simulink model "lab4_S6_7_8_estimation_control_yaw"  (R2024b)
settings: Solver=ode23  StartTime=0.0  StopTime=sIn.simulation_time  RelTol=1e-3
undefined symbols (not defined in the file): chassis, DiscIntNeverNeededParam, drv, feedback, filter, gbox, sens, sIn, wheel
settings Model: Creator=Nihal  LastModifiedBy=pries

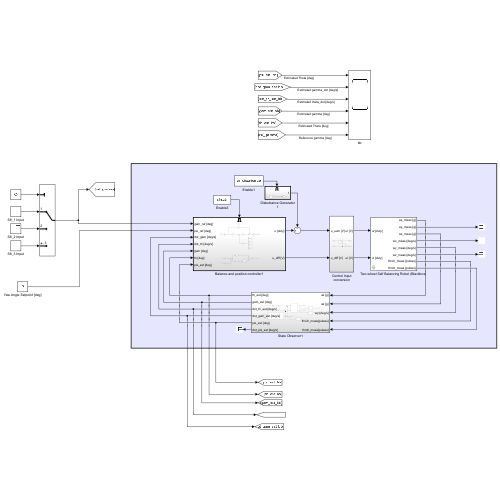
[thumbnail: Simulink's stored preview of the top-level diagram]
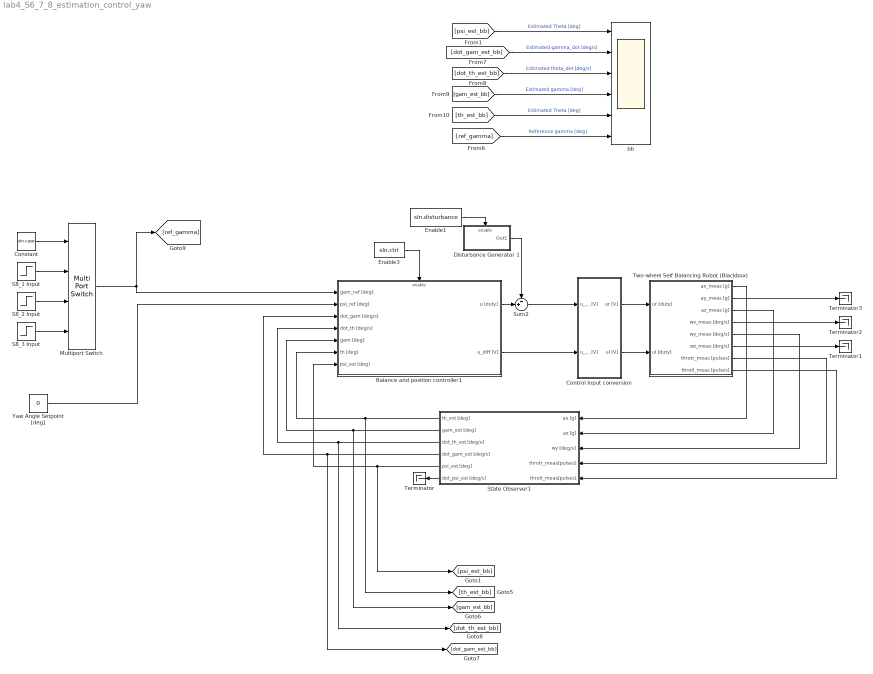
== system lab4_S6_7_8_estimation_control_yaw ==
  Balance and position controller1 : Subsystem
  Constant : Constant  Value=sIn.case
  Control Input conversion : Subsystem
  Disturbance Generator 1 : Subsystem  TreatAsAtomicUnit=on
  Enable1 : Constant  Value=sIn.disturbance
  Enable3 : Constant  Value=sIn.ctrl
  Multiport Switch : MultiPortSwitch  SaturateOnIntegerOverflow=off  InputSameDT=off
  S8_1 Input : Step  Time=0  After=0  SampleTime=0
  S8_2 Input : Step  Time=0  After=(0.1/wheel.r) *rad2deg  SampleTime=0
  S8_3 Input : Step  Time=0  After=(0.1/wheel.r) *rad2deg  SampleTime=0
  State Observer1 : Subsystem
  Sum2 : Sum  Inputs=-+|
  Terminator{,1..3} (4 alike) : Terminator
  "Two-wheel Self Balancing Robot (Blackbox) " : Subsystem  mask(Balancing robot (longitudinal + lateral dynamics)){initState=sIn.bb_ic, Ts=0.01}
      mask prompts: initState "Initial state [gam(0), psi(0), th(0), dot_gam(0), dot_psi(0), dot_th(0)]'"; Ts "Sample time:"
      mask help:
      | Balancing robot dynamic model.
      | Includes both the longitudinal and lateral (yaw) dynamics.
      mask init:
      | %% General parameters and conversion gains
      | 
      | %   gravity acc [m/s^2]
      | g = 9.81;
      | 
      | %   conversion gains
      | rpm2rads = 2*pi/60;         %   [rpm]   -> [rad/s]
      | rads2rpm = 60/2/pi;         %   [rad/s] -> [rpm]
      | rpm2degs = 360/60;          %   [rpm]   -> [deg/s]
      | degs2rpm = 60/360;          %   [deg/s] -> [rpm]
      | deg2rad = pi/180;           %   [deg]   -> [rad]
      | rad2deg = 180/pi;           %   [rad]   -> [deg]
      | g2ms2 = g;                  %   [acc_g] -> [m/s^2]
      | ms22g = 1/g;                %   [m/s^2] -> [acc_g]
      | ozin2Nm = 0.706e-2;         %   [oz*inch] -> [N*m]
      | 
      | 
      | %%  Battery data
      | 
      | %   electrical data
      | batt.UN = 11.1;     %   nominal voltage
      | 
      | 
      | %%  H-bridge PWM voltage driver
      | 
      | drv.Vbus = batt.UN;                     %   H-bridge DC bus voltage  
      | drv.pwm.bits = 8;                       %   PWM resolution [bits]
      | drv.pwm.levels = 2^drv.pwm.bits;        %   PWM levels
      | drv.pwm.Fs = 490;                       %   PWM frequency
      | drv.dutymax = drv.pwm.levels-1;         %   max duty cycle code
      | drv.duty2V = drv.Vbus/drv.dutymax;      %   duty cycle code (0-255) to voltage
      | drv.V2duty = drv.dutymax/drv.Vbus;      %   voltage to duty cycle code (0-255)
      | 
      | 
      | %%  Gearbox data 
      | 
      | gbox.N = 30;            %   reduction ratio
      | 
      | 
      | %%  Sensors data - Hall-effect encoder
      | 
      | %   Hall-effect encoder
      | sens.enc.ppr = 16*4;    %   pulses per rotation at motor side (w/ quadrature decoding)
      | sens.enc.pulse2deg = 360/sens.enc.ppr;
      | sens.enc.pulse2rad = 2*pi/sens.enc.ppr;
      | sens.enc.deg2pulse = sens.enc.ppr/360;
      | sens.enc.rad2pulse = sens.enc.ppr/2/pi;
      | 
      | 
      | %%  Sensors data - MPU6050 (accelerometer + gyro)
      | 
      | %   center of mass (CoM) position
      | sens.mpu.xb = 0;
      | sens.mpu.yb = 0;
      | sens.mpu.zb = 13.5e-3;
      | 
      | %       MPU6050 embedded accelerometer specs
      | sens.mpu.acc.bits = 16;
      | sens.mpu.acc.fs_g = 16;                                                         %   full-scale in "g" units
      | sens.mpu.acc.fs = sens.mpu.acc.fs_g * g2ms2;                                    %   full-scale in [m/s^2] 
      | sens.mpu.acc.g2LSB = floor(2^(sens.mpu.acc.bits-1)/sens.mpu.acc.fs_g);          %   sensitivity [LSB/g]
      | sens.mpu.acc.ms22LSB = sens.mpu.acc.g2LSB * ms22g;                              %   sensitvity [LSB/(m/s^2)]
      | sens.mpu.acc.LSB2g = sens.mpu.acc.fs_g/2^(sens.mpu.acc.bits-1);                 %   output quantization step [g/LSB]
      | sens.mpu.acc.LSB2ms2 = sens.mpu.acc.LSB2g * g2ms2;                              %   output quantization step [ms2/LSB]
      | sens.mpu.acc.bw = 94;                                                           %   output low-pass filter bandwidth
      | sens.mpu.acc.noisestd = 400e-6*sqrt(100);                                       %   output noise std [g-rms]
      | sens.mpu.acc.noisevar = sens.mpu.acc.noisestd^2;                                %   output noise var [g^2]
      | 
      | %       MPU6050 embdedded gyroscope specs
      | sens.mpu.gyro.bits = 16;
      | sens.mpu.gyro.fs_degs = 250;                                                    %   full scale in [deg/s (dps)]
      | sens.mpu.gyro.fs = sens.mpu.gyro.fs_degs * deg2rad;                             %   full scale in [rad/s]
      | sens.mpu.gyro.degs2LSB = floor(2^(sens.mpu.gyro.bits-1)/sens.mpu.gyro.fs_degs);	%   sensitivity [LSB/degs]
      | sens.mpu.gyro.rads2LSB = sens.mpu.gyro.degs2LSB * rad2deg;                      %   sensitivity [LSB/rads] 
      | sens.mpu.gyro.LSB2degs = sens.mpu.gyro.fs_degs/2^(sens.mpu.gyro.bits-1);        %   output quantization step [degs/LSB]
      | sens.mpu.gyro.LSB2rads = sens.mpu.gyro.LSB2degs * deg2rad;                      %   output quantization step [rads/LSB]
      | sens.mpu.gyro.bw = 98;                                                          %   output low-pass filter bandwidth
      | sens.mpu.gyro.noisestd = 5e-3*sqrt(100);                                        %   output noise std [degs-rms]
      | sens.mpu.gyro.noisevar = sens.mpu.acc.noisestd ^2;                              %   output noise var [degs^2]
      mask Help:
      | Riccardo Antonello (antonello@dei.unipd.it)
      | 
      | May 19, 2020
      | 
      | Dept. of Information Engineering, University of Padova
  Yaw Angle Setpoint [deg] : Constant  Value=0
  bb : Scope  NumInputPorts=6
  wires:
  Multiport Switch/1 -> [ref_gamma], Balance and position controller1/1(gam_ref [deg])
  "Two-wheel Self Balancing Robot (Blackbox) "/1(ax_meas [g]) -> State Observer1/1(ax [g])
  "Two-wheel Self Balancing Robot (Blackbox) "/3(az_meas [g]) -> State Observer1/2(az [g])
  "Two-wheel Self Balancing Robot (Blackbox) "/5(wy_meas [deg/s]) -> State Observer1/3(wy [deg/s])
  State Observer1/4(dot_gam_est [deg/s]) -> [dot_gam_est_bb], Balance and position controller1/3(dot_gam [deg/s])
  State Observer1/2(gam_est [deg]) -> [gam_est_bb], Balance and position controller1/5(gam [deg])
  State Observer1/1(th_est [deg]) -> [th_est_bb], Balance and position controller1/6(th [deg])
  State Observer1/3(dot_th_est [deg/s]) -> [dot_th_est_bb], Balance and position controller1/4(dot_th [deg/s])
  [dot_th_est_bb] -> bb/3  "Estimated theta_dot [deg/s]"
  [gam_est_bb] -> bb/4  "Estimated gamma [deg]"
  [ref_gamma] -> bb/6  "Reference gamma [deg]"
  [th_est_bb] -> bb/5  "Estimated Theta [deg]"
  [dot_gam_est_bb] -> bb/2  "Estimated gamma_dot [deg/s]"
  S8_1 Input/1 -> Multiport Switch/2
  S8_2 Input/1 -> Multiport Switch/3
  Constant/1 -> Multiport Switch/1
  S8_3 Input/1 -> Multiport Switch/4
  Enable1/1 -> Disturbance Generator 1/Enable
  Balance and position controller1/1(u [duty]) -> Sum2/2
  Sum2/1 -> Control Input conversion/1(u_sum [V])
  Disturbance Generator 1/1(Out1) -> Sum2/1
  Enable3/1 -> Balance and position controller1/Enable
  State Observer1/5(psi_est [deg]) -> Balance and position controller1/7(psi_est [deg]), [psi_est_bb]
  State Observer1/6(dot_psi_est [deg/s]) -> Terminator/1
  Yaw Angle Setpoint [deg]/1 -> Balance and position controller1/2(psi_ref [deg])
  Control Input conversion/2(ul [V]) -> "Two-wheel Self Balancing Robot (Blackbox) "/2(ul [duty])
  Control Input conversion/1(ur [V]) -> "Two-wheel Self Balancing Robot (Blackbox) "/1(ur [duty])
  Balance and position controller1/2(u_diff [V]) -> Control Input conversion/2(u_diff [V])
  "Two-wheel Self Balancing Robot (Blackbox) "/8(throtl_meas [pulses]) -> State Observer1/5(throtl_meas[pulses])
  "Two-wheel Self Balancing Robot (Blackbox) "/7(throtr_meas [pulses]) -> State Observer1/4(throtr_meas[pulses])
  "Two-wheel Self Balancing Robot (Blackbox) "/6(wz_meas [deg/s]) -> Terminator1/1
  "Two-wheel Self Balancing Robot (Blackbox) "/4(wx_meas [deg/s]) -> Terminator2/1
  "Two-wheel Self Balancing Robot (Blackbox) "/2(ay_meas [g]) -> Terminator3/1
  [psi_est_bb] -> bb/1  "Estimated Theta [deg]"

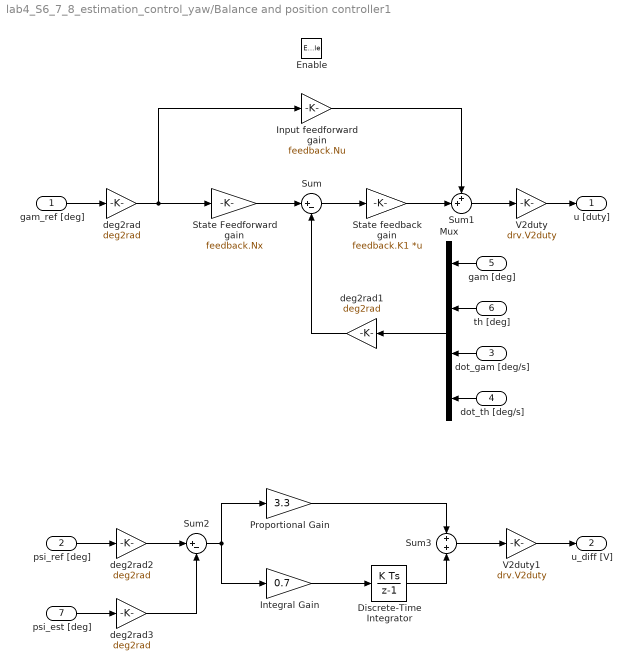
== system lab4_S6_7_8_estimation_control_yaw/Balance and position controller1 ==
  gam_ref [deg] : Inport
  psi_ref [deg] : Inport  Port=2
  dot_gam [deg/s] : Inport  Port=3
  dot_th [deg/s] : Inport  Port=4
  gam [deg] : Inport  Port=5
  th [deg] : Inport  Port=6
  psi_est [deg] : Inport  Port=7
  Enable : EnablePort
  Discrete-Time Integrator : DiscreteIntegrator  SampleTime=-1  ICPrevOutput=DiscIntNeverNeededParam  ICPrevScaledInput=DiscIntNeverNeededParam
  Input feedforward gain : Gain  Gain=feedback.Nu
  Integral Gain : Gain  Gain=0.7
  Mux : Mux
  Proportional Gain : Gain  Gain=3.3
  State Feedforward gain : Gain  Gain=feedback.Nx
  State feedback gain : Gain  Gain=feedback.K1  Multiplication=Matrix(K*u)
  Sum : Sum  Inputs=|+-
  Sum1 : Sum  Inputs=++|
  Sum2 : Sum  Inputs=|+-
  Sum3 : Sum  Inputs=+|+
  V2duty : Gain  Gain=drv.V2duty
  V2duty1 : Gain  Gain=drv.V2duty
  deg2rad{,1..3} (4 alike) : Gain  Gain=deg2rad
  u [duty] : Outport  OutputWhenDisabled=reset  InitialOutput=0
  u_diff [V] : Outport  Port=2  OutputWhenDisabled=reset  InitialOutput=0
  wires:
  gam_ref [deg]/1 -> deg2rad/1
  deg2rad/1 -> Input feedforward gain/1, State Feedforward gain/1
  State Feedforward gain/1 -> Sum/1
  deg2rad1/1 -> Sum/2
  Mux/1 -> deg2rad1/1
  gam [deg]/1 -> Mux/1
  dot_th [deg/s]/1 -> Mux/4
  dot_gam [deg/s]/1 -> Mux/3
  th [deg]/1 -> Mux/2
  Sum/1 -> State feedback gain/1
  State feedback gain/1 -> Sum1/2
  Input feedforward gain/1 -> Sum1/1
  Sum1/1 -> V2duty/1
  V2duty/1 -> u [duty]/1
  psi_ref [deg]/1 -> deg2rad2/1
  psi_est [deg]/1 -> deg2rad3/1
  deg2rad2/1 -> Sum2/1
  deg2rad3/1 -> Sum2/2
  Integral Gain/1 -> Discrete-Time Integrator/1
  Sum2/1 -> Integral Gain/1, Proportional Gain/1
  Proportional Gain/1 -> Sum3/1
  Discrete-Time Integrator/1 -> Sum3/2
  Sum3/1 -> V2duty1/1
  V2duty1/1 -> u_diff [V]/1

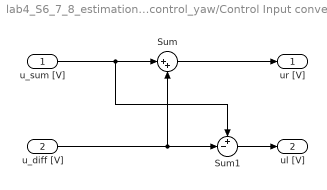
== system lab4_S6_7_8_estimation_control_yaw/Control Input conversion ==
  u_sum [V] : Inport
  u_diff [V] : Inport  Port=2
  Sum : Sum  Inputs=|++
  Sum1 : Sum  Inputs=+-|
  ur [V] : Outport
  ul [V] : Outport  Port=2
  wires:
  u_sum [V]/1 -> Sum/1, Sum1/1
  Sum/1 -> ur [V]/1
  u_diff [V]/1 -> Sum/2, Sum1/2
  Sum1/1 -> ul [V]/1

== system lab4_S6_7_8_estimation_control_yaw/Disturbance Generator 1 ==
  Enable : EnablePort
  Step : Step  Time=10  After=5/drv.duty2V  SampleTime=0
  Out1 : Outport  OutputWhenDisabled=reset  InitialOutput=0
  wires:
  Step/1 -> Out1/1

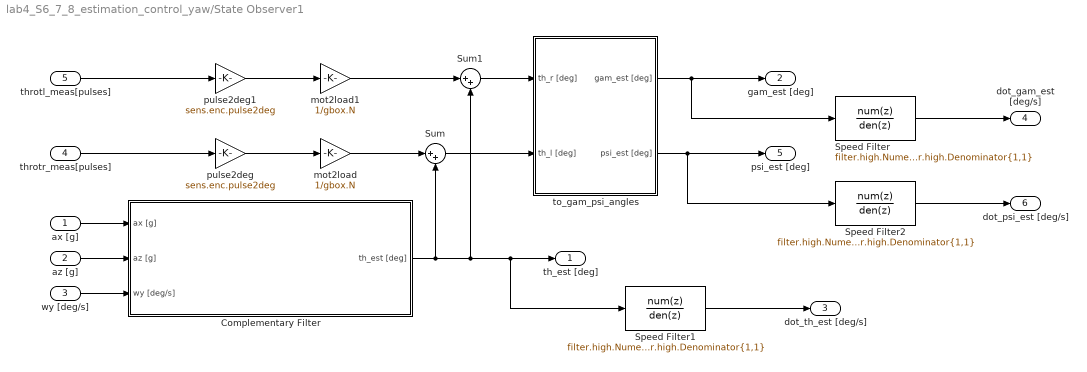
== system lab4_S6_7_8_estimation_control_yaw/State Observer1 ==
  ax [g] : Inport
  az [g] : Inport  Port=2
  wy [deg/s] : Inport  Port=3
  throtr_meas[pulses] : Inport  Port=4
  throtl_meas[pulses] : Inport  Port=5
  Complementary Filter : Subsystem
  Speed Filter : DiscreteFilter  Numerator=filter.high.Numerator{1,1}  Denominator=filter.high.Denominator{1,1}
  Speed Filter1 : DiscreteFilter  Numerator=filter.high.Numerator{1,1}  Denominator=filter.high.Denominator{1,1}
  Speed Filter2 : DiscreteFilter  Numerator=filter.high.Numerator{1,1}  Denominator=filter.high.Denominator{1,1}
  Sum : Sum  Inputs=|++
  Sum1 : Sum  Inputs=|++
  mot2load : Gain  Gain=1/gbox.N
  mot2load1 : Gain  Gain=1/gbox.N
  pulse2deg : Gain  Gain=sens.enc.pulse2deg
  pulse2deg1 : Gain  Gain=sens.enc.pulse2deg
  to_gam_psi_angles : Subsystem
  th_est [deg] : Outport
  gam_est [deg] : Outport  Port=2
  dot_th_est [deg/s] : Outport  Port=3
  dot_gam_est [deg/s] : Outport  Port=4
  psi_est [deg] : Outport  Port=5
  dot_psi_est [deg/s] : Outport  Port=6
  wires:
  wy [deg/s]/1 -> Complementary Filter/3(wy [deg/s])
  az [g]/1 -> Complementary Filter/2(az [g])
  ax [g]/1 -> Complementary Filter/1(ax [g])
  Complementary Filter/1(th_est [deg]) -> Sum/2, Sum1/2, Speed Filter1/1, th_est [deg]/1
  throtr_meas[pulses]/1 -> pulse2deg/1
  pulse2deg/1 -> mot2load/1
  mot2load/1 -> Sum/1
  Speed Filter1/1 -> dot_th_est [deg/s]/1
  Speed Filter/1 -> dot_gam_est [deg/s]/1
  mot2load1/1 -> Sum1/1
  pulse2deg1/1 -> mot2load1/1
  throtl_meas[pulses]/1 -> pulse2deg1/1
  Sum/1 -> to_gam_psi_angles/2(th_l [deg])
  Sum1/1 -> to_gam_psi_angles/1(th_r [deg])
  to_gam_psi_angles/1(gam_est [deg]) -> Speed Filter/1, gam_est [deg]/1
  to_gam_psi_angles/2(psi_est [deg]) -> Speed Filter2/1, psi_est [deg]/1
  Speed Filter2/1 -> dot_psi_est [deg/s]/1

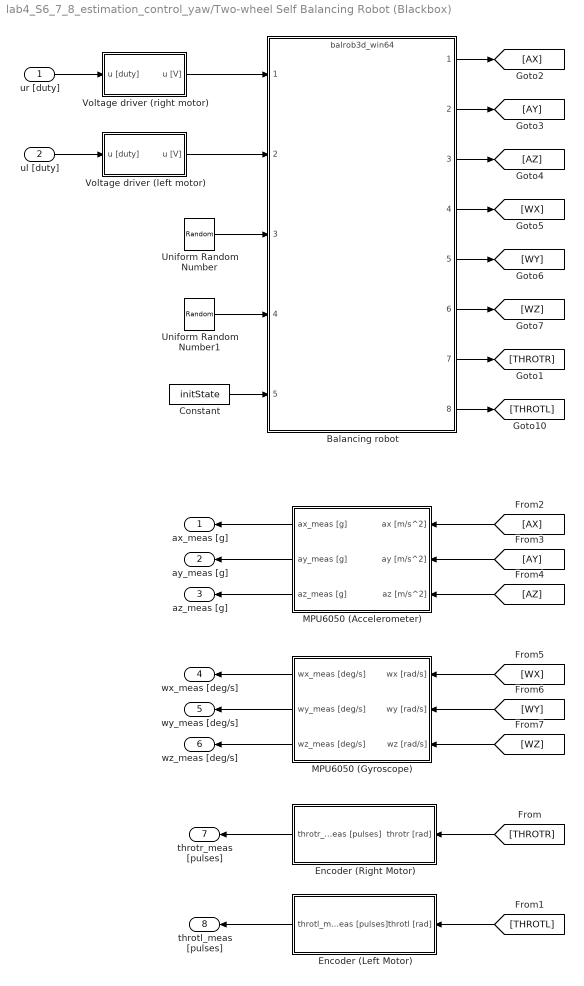
== system lab4_S6_7_8_estimation_control_yaw/Two-wheel Self Balancing Robot (Blackbox)  ==
  ur [duty] : Inport
  ul [duty] : Inport  Port=2
  Balancing robot : ModelReference  ModelNameDialog=balrob3d_win64.slxp  ModelReferenceVersion=1.741  CopyOfModelProtected=on
  Constant : Constant  Value=initState
  Encoder (Left Motor) : Subsystem
  Encoder (Right Motor) : Subsystem
  MPU6050 (Accelerometer) : Subsystem
  MPU6050 (Gyroscope) : Subsystem
  Uniform Random Number : UniformRandomNumber  Minimum=0.7  Maximum=1.3  SampleTime=1
  Uniform Random Number1 : UniformRandomNumber  Minimum=0.7  Maximum=1.3  Seed=10  SampleTime=1
  Voltage driver (left motor) : Subsystem
  Voltage driver (right motor) : Subsystem
  ax_meas [g] : Outport
  ay_meas [g] : Outport  Port=2
  az_meas [g] : Outport  Port=3
  wx_meas [deg/s] : Outport  Port=4
  wy_meas [deg/s] : Outport  Port=5
  wz_meas [deg/s] : Outport  Port=6
  throtr_meas [pulses] : Outport  Port=7
  throtl_meas [pulses] : Outport  Port=8
  wires:
  ur [duty]/1 -> Voltage driver (right motor)/1(u [duty])
  [WX] -> MPU6050 (Gyroscope)/1(wx [rad/s])
  Balancing robot/2 -> [AY]
  Balancing robot/4 -> [WX]
  Balancing robot/8 -> [THROTL]
  Balancing robot/1 -> [AX]
  [THROTL] -> Encoder (Left Motor)/1(throtl [rad])
  Balancing robot/6 -> [WZ]
  Balancing robot/7 -> [THROTR]
  Balancing robot/5 -> [WY]
  [AX] -> MPU6050 (Accelerometer)/1(ax [m/s^2])
  [WY] -> MPU6050 (Gyroscope)/2(wy [rad/s])
  Balancing robot/3 -> [AZ]
  [WZ] -> MPU6050 (Gyroscope)/3(wz [rad/s])
  [AZ] -> MPU6050 (Accelerometer)/3(az [m/s^2])
  [THROTR] -> Encoder (Right Motor)/1(throtr [rad])
  ul [duty]/1 -> Voltage driver (left motor)/1(u [duty])
  [AY] -> MPU6050 (Accelerometer)/2(ay [m/s^2])
  MPU6050 (Accelerometer)/1(ax_meas [g]) -> ax_meas [g]/1
  MPU6050 (Accelerometer)/2(ay_meas [g]) -> ay_meas [g]/1
  MPU6050 (Accelerometer)/3(az_meas [g]) -> az_meas [g]/1
  MPU6050 (Gyroscope)/1(wx_meas [deg/s]) -> wx_meas [deg/s]/1
  MPU6050 (Gyroscope)/2(wy_meas [deg/s]) -> wy_meas [deg/s]/1
  MPU6050 (Gyroscope)/3(wz_meas [deg/s]) -> wz_meas [deg/s]/1
  Encoder (Right Motor)/1(throtr_meas [pulses]) -> throtr_meas [pulses]/1
  Encoder (Left Motor)/1(throtl_meas [pulses]) -> throtl_meas [pulses]/1
  Voltage driver (right motor)/1(u [V]) -> Balancing robot/1
  Voltage driver (left motor)/1(u [V]) -> Balancing robot/2
  Uniform Random Number/1 -> Balancing robot/3
  Uniform Random Number1/1 -> Balancing robot/4
  Constant/1 -> Balancing robot/5

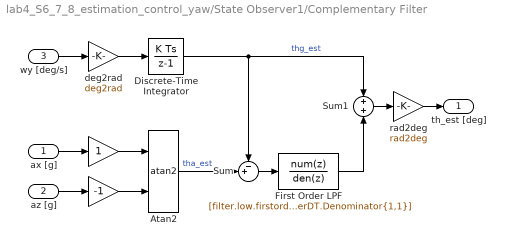
== system lab4_S6_7_8_estimation_control_yaw/State Observer1/Complementary Filter ==
  ax [g] : Inport
  az [g] : Inport  Port=2
  wy [deg/s] : Inport  Port=3
  " " : Gain
  "   " : Gain  Gain=-1
  Atan2 : Trigonometry  Operator=atan2
  Discrete-Time Integrator : DiscreteIntegrator  InitialCondition=sIn.x0(2)  SampleTime=sIn.Ts  ICPrevOutput=DiscIntNeverNeededParam  ICPrevScaledInput=DiscIntNeverNeededParam
  First Order LPF : DiscreteTransferFcn  Numerator=[filter.low.firstorderDT.Numerator{1,1}]  Denominator=[filter.low.firstorderDT.Denominator{1,1}]
  Sum : Sum  Inputs=-+|
  Sum1 : Sum  Inputs=+|+
  deg2rad : Gain  Gain=deg2rad
  rad2deg : Gain  Gain=rad2deg
  th_est [deg] : Outport
  wires:
  wy [deg/s]/1 -> deg2rad/1
  deg2rad/1 -> Discrete-Time Integrator/1
  az [g]/1 -> "   "/1
  ax [g]/1 -> " "/1
  "   "/1 -> Atan2/2
  " "/1 -> Atan2/1
  Atan2/1 -> Sum/2  "tha_est"
  Discrete-Time Integrator/1 -> Sum1/1, Sum/1  "thg_est"
  Sum/1 -> First Order LPF/1
  First Order LPF/1 -> Sum1/2
  Sum1/1 -> rad2deg/1
  rad2deg/1 -> th_est [deg]/1

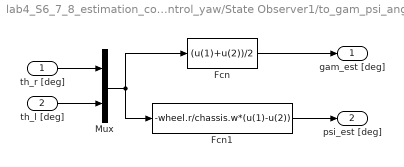
== system lab4_S6_7_8_estimation_control_yaw/State Observer1/to_gam_psi_angles ==
  th_r [deg] : Inport
  th_l [deg] : Inport  Port=2
  Fcn : Fcn  Expr=(u(1)+u(2))/2
  Fcn1 : Fcn  Expr=-wheel.r/chassis.w*(u(1)-u(2))
  Mux : Mux  Inputs=2
  gam_est [deg] : Outport
  psi_est [deg] : Outport  Port=2
  wires:
  th_r [deg]/1 -> Mux/1
  th_l [deg]/1 -> Mux/2
  Mux/1 -> Fcn1/1, Fcn/1
  Fcn/1 -> gam_est [deg]/1
  Fcn1/1 -> psi_est [deg]/1

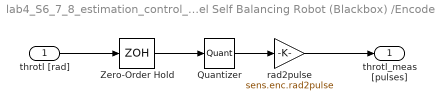
== system lab4_S6_7_8_estimation_control_yaw/Two-wheel Self Balancing Robot (Blackbox) /Encoder (Left Motor) ==
  throtl [rad] : Inport
  Quantizer : Quantizer  QuantizationInterval=sens.enc.pulse2rad
  Zero-Order Hold : ZeroOrderHold  SampleTime=Ts
  rad2pulse : Gain  Gain=sens.enc.rad2pulse
  throtl_meas [pulses] : Outport
  wires:
  Quantizer/1 -> rad2pulse/1
  Zero-Order Hold/1 -> Quantizer/1
  throtl [rad]/1 -> Zero-Order Hold/1
  rad2pulse/1 -> throtl_meas [pulses]/1

== system lab4_S6_7_8_estimation_control_yaw/Two-wheel Self Balancing Robot (Blackbox) /Encoder (Right Motor) ==
  throtr [rad] : Inport
  Quantizer : Quantizer  QuantizationInterval=sens.enc.pulse2rad
  Zero-Order Hold : ZeroOrderHold  SampleTime=Ts
  rad2pulse : Gain  Gain=sens.enc.rad2pulse
  throtr_meas [pulses] : Outport
  wires:
  throtr [rad]/1 -> Zero-Order Hold/1
  Zero-Order Hold/1 -> Quantizer/1
  Quantizer/1 -> rad2pulse/1
  rad2pulse/1 -> throtr_meas [pulses]/1

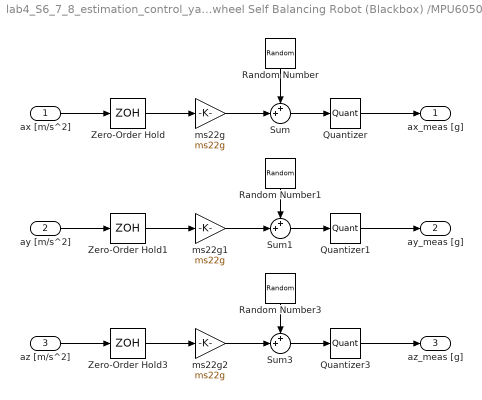
== system lab4_S6_7_8_estimation_control_yaw/Two-wheel Self Balancing Robot (Blackbox) /MPU6050 (Accelerometer) ==
  ax [m/s^2] : Inport
  ay [m/s^2] : Inport  Port=2
  az [m/s^2] : Inport  Port=3
  Quantizer : Quantizer  QuantizationInterval=sens.mpu.acc.LSB2g
  Quantizer1 : Quantizer  QuantizationInterval=sens.mpu.acc.LSB2g
  Quantizer3 : Quantizer  QuantizationInterval=sens.mpu.acc.LSB2g
  Random Number : RandomNumber  Variance=sens.mpu.acc.noisevar  Seed=1  SampleTime=Ts
  Random Number1 : RandomNumber  Variance=sens.mpu.acc.noisevar  Seed=10  SampleTime=Ts
  Random Number3 : RandomNumber  Variance=sens.mpu.acc.noisevar  Seed=100  SampleTime=Ts
  Sum : Sum  Inputs=++|
  Sum1 : Sum  Inputs=++|
  Sum3 : Sum  Inputs=++|
  Zero-Order Hold : ZeroOrderHold  SampleTime=Ts
  Zero-Order Hold1 : ZeroOrderHold  SampleTime=Ts
  Zero-Order Hold3 : ZeroOrderHold  SampleTime=Ts
  ms22g : Gain  Gain=ms22g
  ms22g1 : Gain  Gain=ms22g
  ms22g2 : Gain  Gain=ms22g
  ax_meas [g] : Outport
  ay_meas [g] : Outport  Port=2
  az_meas [g] : Outport  Port=3
  wires:
  ax [m/s^2]/1 -> Zero-Order Hold/1
  Zero-Order Hold1/1 -> ms22g1/1
  Sum1/1 -> Quantizer1/1
  ms22g/1 -> Sum/2
  ay [m/s^2]/1 -> Zero-Order Hold1/1
  Sum3/1 -> Quantizer3/1
  ms22g1/1 -> Sum1/2
  Random Number1/1 -> Sum1/1
  Random Number/1 -> Sum/1
  Sum/1 -> Quantizer/1
  Random Number3/1 -> Sum3/1
  ms22g2/1 -> Sum3/2
  Zero-Order Hold3/1 -> ms22g2/1
  az [m/s^2]/1 -> Zero-Order Hold3/1
  Zero-Order Hold/1 -> ms22g/1
  Quantizer/1 -> ax_meas [g]/1
  Quantizer1/1 -> ay_meas [g]/1
  Quantizer3/1 -> az_meas [g]/1

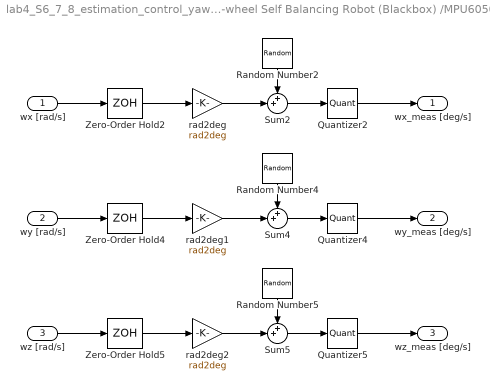
== system lab4_S6_7_8_estimation_control_yaw/Two-wheel Self Balancing Robot (Blackbox) /MPU6050 (Gyroscope) ==
  wx [rad/s] : Inport
  wy [rad/s] : Inport  Port=2
  wz [rad/s] : Inport  Port=3
  Quantizer2 : Quantizer  QuantizationInterval=sens.mpu.gyro.LSB2degs
  Quantizer4 : Quantizer  QuantizationInterval=sens.mpu.gyro.LSB2degs
  Quantizer5 : Quantizer  QuantizationInterval=sens.mpu.gyro.LSB2degs
  Random Number2 : RandomNumber  Variance=sens.mpu.gyro.noisevar  Seed=2  SampleTime=Ts
  Random Number4 : RandomNumber  Variance=sens.mpu.gyro.noisevar  Seed=20  SampleTime=Ts
  Random Number5 : RandomNumber  Variance=sens.mpu.gyro.noisevar  Seed=200  SampleTime=Ts
  Sum2 : Sum  Inputs=++|
  Sum4 : Sum  Inputs=++|
  Sum5 : Sum  Inputs=++|
  Zero-Order Hold2 : ZeroOrderHold  SampleTime=Ts
  Zero-Order Hold4 : ZeroOrderHold  SampleTime=Ts
  Zero-Order Hold5 : ZeroOrderHold  SampleTime=Ts
  rad2deg : Gain  Gain=rad2deg
  rad2deg1 : Gain  Gain=rad2deg
  rad2deg2 : Gain  Gain=rad2deg
  wx_meas [deg/s] : Outport
  wy_meas [deg/s] : Outport  Port=2
  wz_meas [deg/s] : Outport  Port=3
  wires:
  Random Number2/1 -> Sum2/1
  Sum2/1 -> Quantizer2/1
  Quantizer2/1 -> wx_meas [deg/s]/1
  Zero-Order Hold5/1 -> rad2deg2/1
  Sum4/1 -> Quantizer4/1
  rad2deg/1 -> Sum2/2
  rad2deg2/1 -> Sum5/2
  Random Number5/1 -> Sum5/1
  Zero-Order Hold4/1 -> rad2deg1/1
  Sum5/1 -> Quantizer5/1
  Random Number4/1 -> Sum4/1
  Zero-Order Hold2/1 -> rad2deg/1
  Quantizer5/1 -> wz_meas [deg/s]/1
  wz [rad/s]/1 -> Zero-Order Hold5/1
  wx [rad/s]/1 -> Zero-Order Hold2/1
  rad2deg1/1 -> Sum4/2
  Quantizer4/1 -> wy_meas [deg/s]/1
  wy [rad/s]/1 -> Zero-Order Hold4/1

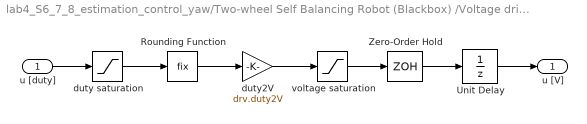
== system lab4_S6_7_8_estimation_control_yaw/Two-wheel Self Balancing Robot (Blackbox) /Voltage driver (left motor) ==
  u [duty] : Inport
  Rounding Function : Rounding  Operator=fix
  Unit Delay : UnitDelay  SampleTime=1/drv.pwm.Fs  HasFrameUpgradeWarning=on
  Zero-Order Hold : ZeroOrderHold  SampleTime=Ts
  duty saturation : Saturate  UpperLimit=255  LowerLimit=-255
  duty2V : Gain  Gain=drv.duty2V
  voltage saturation : Saturate  UpperLimit=drv.Vbus  LowerLimit=-drv.Vbus
  u [V] : Outport
  wires:
  Zero-Order Hold/1 -> Unit Delay/1
  u [duty]/1 -> duty saturation/1
  voltage saturation/1 -> Zero-Order Hold/1
  duty saturation/1 -> Rounding Function/1
  Rounding Function/1 -> duty2V/1
  duty2V/1 -> voltage saturation/1
  Unit Delay/1 -> u [V]/1

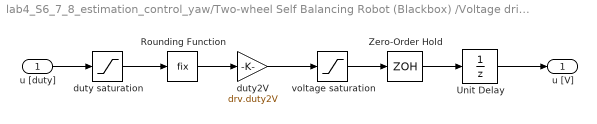
== system lab4_S6_7_8_estimation_control_yaw/Two-wheel Self Balancing Robot (Blackbox) /Voltage driver (right motor) ==
  u [duty] : Inport
  Rounding Function : Rounding  Operator=fix
  Unit Delay : UnitDelay  SampleTime=1/drv.pwm.Fs  HasFrameUpgradeWarning=on
  Zero-Order Hold : ZeroOrderHold  SampleTime=Ts
  duty saturation : Saturate  UpperLimit=255  LowerLimit=-255
  duty2V : Gain  Gain=drv.duty2V
  voltage saturation : Saturate  UpperLimit=drv.Vbus  LowerLimit=-drv.Vbus
  u [V] : Outport
  wires:
  u [duty]/1 -> duty saturation/1
  duty saturation/1 -> Rounding Function/1
  Zero-Order Hold/1 -> Unit Delay/1
  voltage saturation/1 -> Zero-Order Hold/1
  Rounding Function/1 -> duty2V/1
  duty2V/1 -> voltage saturation/1
  Unit Delay/1 -> u [V]/1
